simulink model "EKF"  (R2024a)
settings: Solver=FixedStepAuto  StartTime=0.0  StopTime=15  FixedStep=Ts  RelTol=1e-3
values from neighbouring files (symbols this model uses):
  Ts = 0.001    [AFEKF.m]    (also in DCMotorJacobianFcn.m; EKF_J_D.m = 0.005)
settings Model: Creator=rocke  LastModifiedBy=rocke

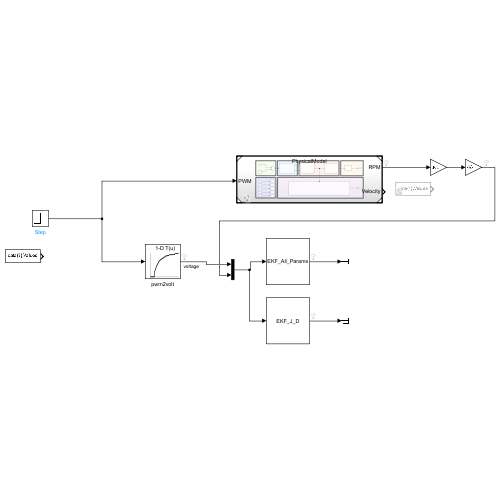
[thumbnail: Simulink's stored preview of the top-level diagram]
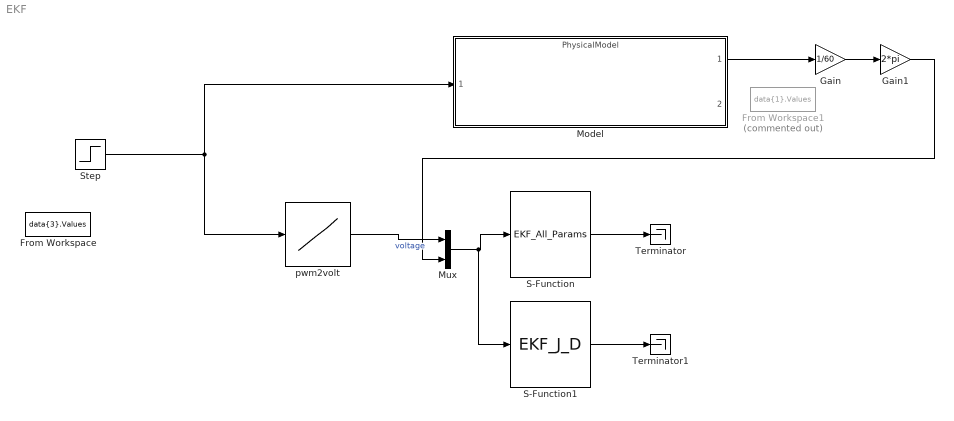
== system EKF ==
  From Workspace : FromWorkspace  VariableName=data{3}.Values  SampleTime=-1
  From Workspace1 : FromWorkspace  Commented=on  VariableName=data{1}.Values  SampleTime=-1
  Gain : Gain  Gain=1/60
  Gain1 : Gain  Gain=2*pi
  Model : ModelReference  ModelNameDialog=PhysicalModel.slx  SimulationMode=Normal  ModelReferenceVersion=1.28
  Mux : Mux  Inputs=2
  S-Function : S-Function  FunctionName=EKF_All_Params  SFunctionDeploymentMode=off  EnableBusSupport=off
  S-Function1 : S-Function  FunctionName=EKF_J_D  SFunctionDeploymentMode=off  EnableBusSupport=off
  Step : Step  After=155  SampleTime=Ts
  Terminator : Terminator
  Terminator1 : Terminator
  pwm2volt : Lookup_n-D  NumberOfTableDimensions=1  BreakpointsForDimension1=[0 5 10 15 20 25 30 35 40 45 50 55 60 65 70 75 80 85 90 95 100 105 110 115 120 125 130 135 140 145 150 155 160 165 170 175 180 185 190 195 200 205 210 215 220 225 230 235 240 245 250 255]  Table=[0;0;0;0;0;0;0;0;2.5;3.08;3.77;4.54;5.08;5.55;6.05;6.5;6.97;7.23;7.51;7.72;7.9;8.09;8.28;8.4;8.56;8.65;8.87;9.07;9.27;9.33;9.45;9.51;9.59;9.66;9.74;9.82;9.89;9.91;9.96;10.04;10.08;10.11;10.14;10.2;10.26;10.31;10.37;10.43;10.47;10.47;10.52;10.74]  InternalRulePriority=Speed  RndMeth=Simplest
  wires:
  pwm2volt/1 -> Mux/1  "voltage"
  Step/1 -> pwm2volt/1, Model/1
  Gain/1 -> Gain1/1
  Gain1/1 -> Mux/2
  Mux/1 -> S-Function1/1, S-Function/1
  S-Function/1 -> Terminator/1
  S-Function1/1 -> Terminator1/1
  Model/1 -> Gain/1
